simulink model "Controllers_deimian"  (R2023a)
settings: Solver=VariableStepAuto  StartTime=0.0  StopTime=10  RelTol=1e-3
values from neighbouring files (symbols this model uses):
  Gpz_den = Gpz.Denominator{1,1}    [deimian.m]
  Gpz_num = Gpz.Numerator{1,1}    [deimian.m]
  Kdz = (Kp*Taud)/T    (= 62.7240538515)    [deimian.m]
  Kiz = (Kp*T)/Taui    (= 42.7148147579)    [deimian.m]
  Kpz = Kp - (Kp * T)/(2*Taui)    (= 144.229508103)    [deimian.m]
  T = 0.05    [deimian.m]
undefined symbols (not defined in the file or in its folder): DiscIntNeverNeededParam
libraries: simulink x1
settings Model: Creator=maxpr  LastModifiedBy=maxpr

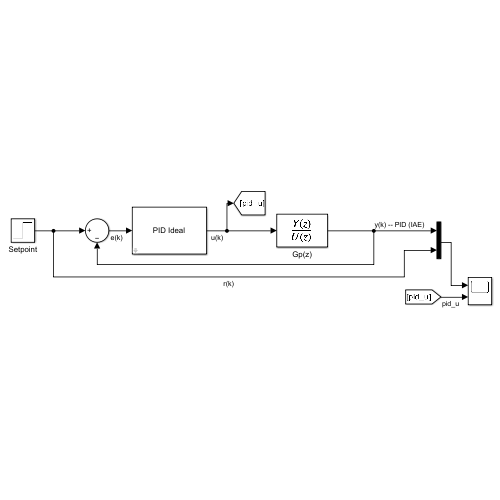
[thumbnail: Simulink's stored preview of the top-level diagram]
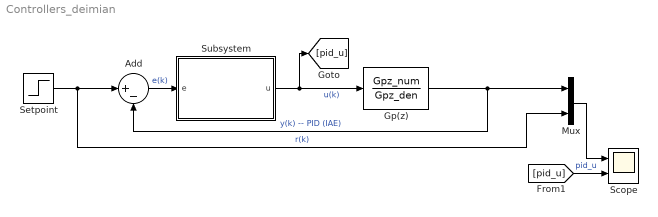
== system Controllers_deimian ==
  Add : Sum  Inputs=|+-
  Gp(z) : DiscreteTransferFcn  Numerator=Gpz_num  Denominator=Gpz_den  SampleTime=T
  Mux : Mux  Inputs=2
  Scope : Scope  NumInputPorts=2
  Setpoint : Step  After=1.5  SampleTime=T
  Subsystem : Subsystem  mask{Kp=Kpz, Ki=Kiz, Kd=Kdz}
      mask prompts: Kp "Ganancia proporcional"; Ki "Ganancia integral"; Kd "Ganancia derivativa"
      mask DialogControl ParameterGroupVar Prompt: PID params
      mask Display: disp('PID Ideal');
  wires:
  Add/1 -> Subsystem/1(e)  "e(k)"
  Subsystem/1(u) -> [pid_u], Gp(z)/1  "u(k)"
  Gp(z)/1 -> Mux/1, Add/2  "y(k) -- PID (IAE)"
  Mux/1 -> Scope/1
  [pid_u] -> Scope/2  "pid_u"
  Setpoint/1 -> Mux/2, Add/1  "r(k)"

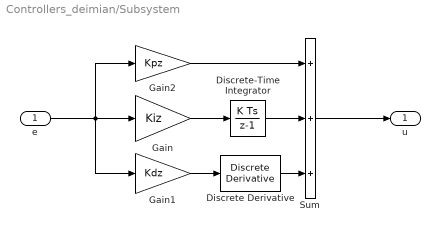
== system Controllers_deimian/Subsystem ==
  e : Inport
  Discrete Derivative : simulink/Discrete/Discrete Derivative  gainval=1.0  ICPrevScaledInput=0.0  OutMin=[]  OutMax=[]  OutDataType=fixdt(1, 16)  OutScaling=2^-10  DoSatur=off
  Discrete-Time Integrator : DiscreteIntegrator  SampleTime=T  ICPrevOutput=DiscIntNeverNeededParam  ICPrevScaledInput=DiscIntNeverNeededParam
  Gain : Gain  Gain=Kiz
  Gain1 : Gain  Gain=Kdz
  Gain2 : Gain  Gain=Kpz
  Sum : Sum  Inputs=+++
  u : Outport
  wires:
  e/1 -> Gain1/1, Gain/1, Gain2/1
  Sum/1 -> u/1
  Gain/1 -> Discrete-Time Integrator/1
  Gain1/1 -> Discrete Derivative/1
  Discrete Derivative/1 -> Sum/3
  Gain2/1 -> Sum/1
  Discrete-Time Integrator/1 -> Sum/2
